simulink model "sns_bridge_cpg"  (R2025a)
settings: Solver=ode1  StartTime=0.0  StopTime=5  FixedStep=0.002  RelTol=1e-3
undefined symbols (not defined in the file or in its folder): uvec
libraries: mjLib x1
settings Model: Creator=Ben Bolen  LastModifiedBy=Ben Bolen
settings DataIOCC: SignalLoggingName=sigs

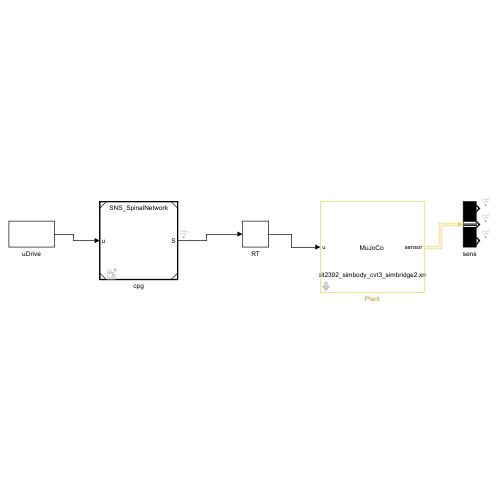
[thumbnail: Simulink's stored preview of the top-level diagram]
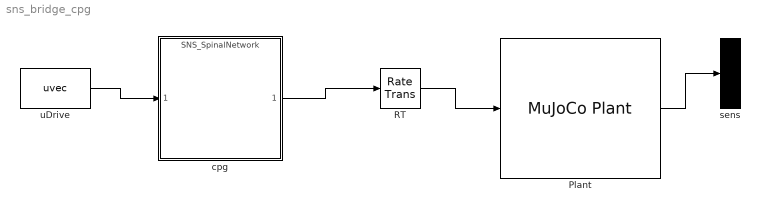
== system sns_bridge_cpg ==
  Plant : mjLib/MuJoCo Plant  controlBus=[]  sensorBus=mj_bus_sensor_7979902499018342666  controlLength=[]  sensorLength=[]  rgbLength=[]  depthLength=[]  sampleTime=0.002  xmlFileRel=D:/Github/Bipedal_Robot/Code/Matlab/SNS_Simscape/mujoco_bridge/matlab/../../../../../Solid_Models/OpenSim/Gait2392_Robotbody/mjc/gait2392_simbody/gait2392_simbody_cvt3_simbridge2.xml  xmlFile=D:/Github/Bipedal_Robot/Code/Matlab/SNS_Simscape/mujoco_bridge/matlab/../../../../../Solid_Models/OpenSim/Gait2392_Robotbody/mjc/gait2392_simbody/gait2392_simbody_cvt3_simbridge2.xml  renderingType=None  vsync=off  visualFPS=60  zoomLevel=1  znear=0.02  zfar=100  cameraSampleTime=0.020  rgbOutOption=off  depthOutOption=off  controlInterfaceType=Vector
      settings: SourceProductName=MuJoCo Simulator
  RT : RateTransition
  cpg : ModelReference  ModelNameDialog=SNS_SpinalNetwork.slx  SimulationMode=Normal  ModelReferenceVersion=1.2
  sens : BusSelector  OutputSignals=knee_r_pos,vas_med_r_len,vas_med_r_frc
  uDrive : Constant  Value=uvec
  wires:
  uDrive/1 -> cpg/1
  cpg/1 -> RT/1
  RT/1 -> Plant/1
  Plant/1 -> sens/1
